simulink model "PID_reg"  (R2018a)
settings: Solver=VariableStepAuto  StartTime=0.0  StopTime=10.0  RelTol=1e-3
values from neighbouring files (symbols this model uses):
  D = 70e-3    (= 0.07)    [HPS.m]
  I = Kp/Ti    (= 4800)    [HPS.m]
  Kp = 0.6*Kkr    (= 84)    [HPS.m]
settings Model: Creator=test4  LastModifiedBy=test4

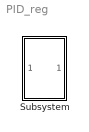
== system PID_reg ==
  Subsystem : Subsystem

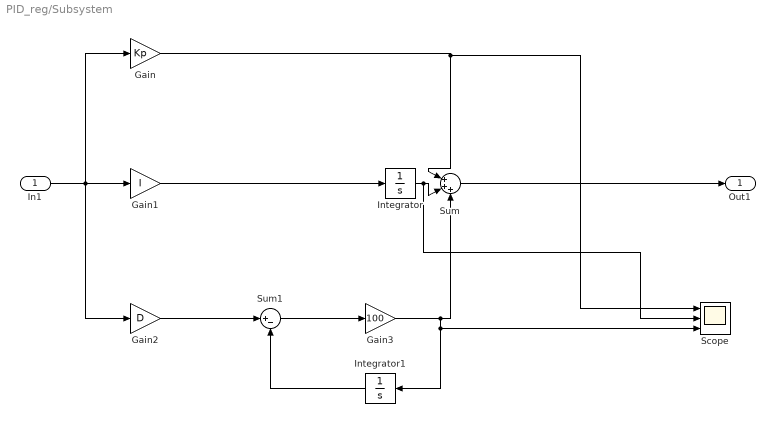
== system PID_reg/Subsystem ==
  In1 : Inport
  Gain : Gain  Gain=Kp
  Gain1 : Gain  Gain=I
  Gain2 : Gain  Gain=D
  Gain3 : Gain  Gain=100
  Integrator : Integrator
  Integrator1 : Integrator
  Scope : Scope  NumInputPorts=3
  Sum : Sum  Inputs=|+++
  Sum1 : Sum  Inputs=|+-
  Out1 : Outport
  wires:
  Gain3/1 -> Scope/3, Integrator1/1, Sum/3
  Integrator/1 -> Scope/2, Sum/2
  Gain2/1 -> Sum1/1
  In1/1 -> Gain2/1, Gain1/1, Gain/1
  Sum/1 -> Out1/1
  Sum1/1 -> Gain3/1
  Gain1/1 -> Integrator/1
  Integrator1/1 -> Sum1/2
  Gain/1 -> Scope/1, Sum/1
